simulink model "collection_of_systems_draft"  (R2022b)
settings: Solver=VariableStepAuto  StartTime=0.0  StopTime=15  RelTol=1e-3
values from neighbouring files (symbols this model uses):
  lbu_body = repmat(srbd_model_obj.input_constraints(:,1),Nb,1)    [initialize_sim_parameters.m]
  lbu_leg = repmat(leg_model_obj.input_constraints(:,1),Nl,1)    [initialize_sim_parameters.m]    (also in pos_control_setup.m)
  lbx_leg = repmat(leg_model_obj.state_constraints(:,1),Nl-1,1)    [initialize_sim_parameters.m]    (also in pos_control_setup.m)
  lg_leg = repmat(lower_g,Nl,1)    [initialize_sim_parameters.m]    (also in pos_control_setup.m)
  lh_e_leg = [0;0]    [initialize_sim_parameters.m]    (also in pos_control_setup.m)
  lh_leg = repmat([0;0],Nl,1)    [initialize_sim_parameters.m]    (also in pos_control_setup.m)
  Nb = 50    [initialize_sim_parameters.m]
  Nl = 5    [initialize_sim_parameters.m]    (also in pos_control_setup.m = 30)
  nu_b = 3    [initialize_sim_parameters.m]
  nu_l = 3    [initialize_sim_parameters.m]    (also in pos_control_setup.m)
  nx_b = 7    [initialize_sim_parameters.m]
  Rinterface = eul2rotm([0,0,-pi/2])    [initialize_sim_parameters.m]
  sampling_body = 2e-2    (= 0.02)    [initialize_sim_parameters.m]
  Thb = 5    [initialize_sim_parameters.m]
  Thl = 0.1    [initialize_sim_parameters.m]    (also in sim_report.m = 0.2)
  ubu_body = repmat(srbd_model_obj.input_constraints(:,2),Nb,1)    [initialize_sim_parameters.m]
  ubu_leg = repmat(leg_model_obj.input_constraints(:,2),Nl,1)    [initialize_sim_parameters.m]    (also in pos_control_setup.m)
  ubx_leg = repmat(leg_model_obj.state_constraints(:,2),Nl-1,1)    [initialize_sim_parameters.m]    (also in pos_control_setup.m)
  ug_leg = repmat(upper_g,Nl,1)    [initialize_sim_parameters.m]    (also in pos_control_setup.m)
  uh_e_leg = [0;0]    [initialize_sim_parameters.m]    (also in pos_control_setup.m)
  uh_leg = repmat([0;0],Nl,1)    [initialize_sim_parameters.m]    (also in pos_control_setup.m)
  y_ref_body = repmat(yref_body,Nb-1,1)    [initialize_sim_parameters.m]
  yref_body = [Qc,zeros(nx_b,nu_b);zeros(nu_b,nx_b),Rc]*[xref_b;0;0;0]    [initialize_sim_parameters.m]
settings Model: Creator=papaveneti  LastModifiedBy=papaveneti

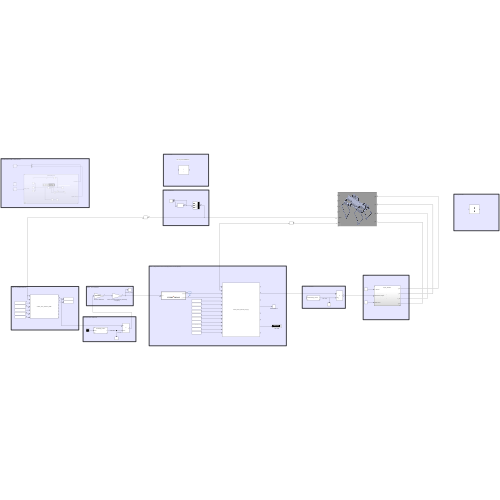
[thumbnail: Simulink's stored preview of the top-level diagram]
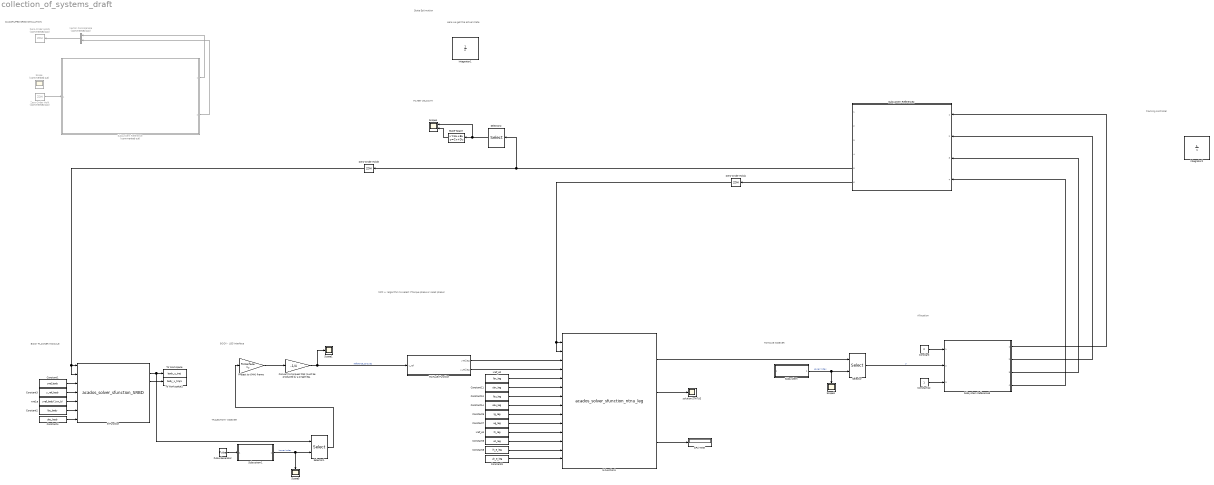
== system collection_of_systems_draft ==
  note: TORQUE INDEXER
  note: TRAJECTORY INDEXER
  note: FILTER VELOCITY
  note: Here we get the actual state
  note: tracking controller
  note: Allocation
  note: MPC + (algorithm to select if torque phase or reset phase)
  note: BODY - LEG interface
  note: QUADRUPED SRBD SIMULATION
  note: BODY PLANNER MODULE
  note: State Estimation
  CPU TIME : Display
  Constant : Constant  Value=0
  Constant1 : Constant  Value=yref_body
  Constant11 : Constant  Value=ubx_leg
  Constant12 : Constant
  Constant13 : Constant  Value=lbu_leg
  Constant14 : Constant  Value=ubu_leg
  Constant2 : Constant  Value=lbu_body
  Constant3 : Constant  Value=y_ref_body
  Constant4 : Constant  Value=ubu_body
  Constant5 : Constant  Value=lg_leg
  Constant6 : Constant  Value=uh_leg
  Constant7 : Constant  Value=ug_leg
  Constant8 : Constant  Value=lh_e_leg
  Constant9 : Constant  Value=uh_e_leg
  Convert to torques that must be produced by a single leg. : Gain  Gain=-1/4
  Integrator1 : Integrator
  Integrator2 : Integrator
  MATLAB Function : MATLAB Function  TreatAsAtomicUnit=on
  "Project to {MH} frame" : Gain  Gain=Rinterface  Multiplication=Matrix(K*u)
  Pulse Generator : DiscretePulseGenerator  PulseType=Time based  Period=1  PulseWidth=5  PhaseDelay=1
  S-Function : S-Function  FunctionName=acados_solver_sfunction_SRBD  SFunctionDeploymentMode=off  EnableBusSupport=off
  S-Function1 : S-Function  FunctionName=acados_solver_sfunction_ntnu_leg  SFunctionDeploymentMode=off  EnableBusSupport=off
  Scope : Scope  Commented=on
  Scope1 : Scope
  Scope3 : Scope
  Scope4 : Scope  NumInputPorts=2
  Scope5 : Scope
  Selector : Selector  InputPortWidth=Nl*nu_l  IndexOptions=Starting index (port)  Indices=[1 3]  OutputSizes=nu_l
  Selector1 : Selector  InputPortWidth=nu_b*Nb  IndexOptions=Starting index (port)  Indices=[1 3]  OutputSizes=nu_l
  Selector2 : Selector  InputPortWidth=7  IndexOptions=Index vector (dialog)  Indices=[5:7]  OutputSizes=1
  State-Space : StateSpace  A=diag([-5,-5,-5])  B=2*eye(3)  C=2.5*eye(3)  D=zeros(3,3)  InitialCondition=0
  Subsystem : Subsystem  ReferencedSubsystem=overflowing_counter  Td=Thl/Nl  Overflow_point=nu_l*Nl  Increment=nu_l
  Subsystem Reference : Subsystem  Commented=on  ReferencedSubsystem=quadruped_base
  Subsystem Reference2 : Subsystem  ReferencedSubsystem=olympus
  Subsystem Reference3 : Subsystem  ReferencedSubsystem=torque_allocation
  Subsystem1 : Subsystem  ReferencedSubsystem=overflowing_counter  Td=Thb/Nb  Overflow_point=nu_b*Nb  Increment=nu_b
  To Workspace : ToWorkspace  VariableName=body_u_traj  SaveFormat=Timeseries  SampleTime=-1
  To Workspace1 : ToWorkspace  VariableName=body_x_traj1  SaveFormat=Timeseries  SampleTime=-1
  Vector Concatenate : Concatenate  Commented=on
  Zero-Order Hold : ZeroOrderHold  Commented=on  SampleTime=sampling_body
  Zero-Order Hold1 : ZeroOrderHold  Commented=on  SampleTime=sampling_body
  Zero-Order Hold3 : ZeroOrderHold
  Zero-Order Hold4 : ZeroOrderHold  SampleTime=Thl/Nl
  solution STATUS : Scope
  xref_e : Constant  Value=yref_body(1:nx_b)
  xref_e1 : Constant  Value=lh_leg
  xref_e2 : Constant  Value=lbx_leg
  wires:
  Zero-Order Hold/1 -> Subsystem Reference/1
  Subsystem Reference/1 -> Vector Concatenate/1
  Subsystem Reference/2 -> Vector Concatenate/2
  Vector Concatenate/1 -> Zero-Order Hold1/1
  S-Function/2 -> Selector1/1, To Workspace/1
  S-Function/3 -> To Workspace1/1
  Constant2/1 -> S-Function/6
  xref_e/1 -> S-Function/5
  Constant4/1 -> S-Function/7
  Constant3/1 -> S-Function/4
  Constant1/1 -> S-Function/3
  "Project to {MH} frame"/1 -> Convert to torques that must be produced by a single leg./1
  Convert to torques that must be produced by a single leg./1 -> MATLAB Function/1(u_ref), Scope1/1  "reference_torques"
  Constant7/1 -> S-Function1/10
  xref_e1/1 -> S-Function1/11
  Constant6/1 -> S-Function1/12
  Constant8/1 -> S-Function1/13
  Constant9/1 -> S-Function1/14
  Constant5/1 -> S-Function1/9
  Constant14/1 -> S-Function1/8
  Constant13/1 -> S-Function1/7
  Constant11/1 -> S-Function1/6
  xref_e2/1 -> S-Function1/5
  MATLAB Function/2(y_ref_leg) -> S-Function1/4
  S-Function1/7 -> CPU TIME/1
  MATLAB Function/1(yref_leg) -> S-Function1/3
  S-Function1/2 -> Selector/1
  Selector/1 -> Subsystem Reference3/2  "U"
  Subsystem/1 -> Selector/2, Scope3/1  "Lower Index"
  S-Function1/4 -> solution STATUS/1
  Subsystem Reference3/1 -> Subsystem Reference2/1
  Subsystem Reference3/2 -> Subsystem Reference2/2
  Subsystem Reference3/3 -> Subsystem Reference2/3
  Subsystem Reference3/4 -> Subsystem Reference2/4
  Subsystem Reference2/5 -> Selector2/1, Zero-Order Hold3/1
  Zero-Order Hold3/1 -> S-Function/2, S-Function/1
  Subsystem Reference2/6 -> Zero-Order Hold4/1
  Zero-Order Hold4/1 -> S-Function1/2, S-Function1/1
  Constant/1 -> Subsystem Reference3/1
  Constant12/1 -> Subsystem Reference3/3
  Subsystem1/1 -> Scope5/1, Selector1/2  "Lower Index"
  Selector2/1 -> State-Space/1, Scope4/1
  State-Space/1 -> Scope4/2
  Selector1/1 -> "Project to {MH} frame"/1
  Pulse Generator/1 -> Subsystem1/1

== matlab function collection_of_systems_draft/MATLAB Function ==
  data: u_ref input size=3; yref_leg output; y_ref_leg output double size=24; Nl parameter size=1
function [yref_leg,y_ref_leg] = REFERENCE_GENERATOR(u_ref,Nl)

tau_mh_ref = u_ref;
torque_reference = [0;0];
constr_ref = 0;

y_ref_leg          = zeros(24,1);
yref_leg           = [tau_mh_ref ; torque_reference; constr_ref];
y_ref_leg(1:24,1)  = repmat(yref_leg,Nl-1,1);
